simulink model "XMC_FFT2D_HLS_AIE"  (R2024a)
settings: Solver=VariableStepAuto  StartTime=0.0  StopTime=256*256*2  RelTol=1e-3
PreLoadFcn:
  | % display k space image & load arrays for
  | % simulation run
  | MRIDemo_PreloadFcn;
undefined symbols (not defined in the file): gray, None, S, vsva2197, xcvc1902
libraries: aieDSP x2, dspxfrm3 x2, dspsrcs4 x2, hlsBasic x1, simulink x1, vmcUtilities x1, aieUtilities x1
settings Model: Creator=mmi  LastModifiedBy=robg
settings SolverCC: AlgebraicLoopSolver=TrustRegion
settings DataIOCC: ReturnWorkspaceOutputs=off
settings DebuggingCC: UnconnectedInputMsg=warning  UnconnectedOutputMsg=warning  UnconnectedLineMsg=warning  ArithmeticOperatorsInVariantConditions=warning
settings ModelReferenceCC: EnableRefExpFcnMdlSchedulingChecks=on
settings SFSimCC: SimUseLocalCustomCode=off  CustomCodeUndefinedFunction=UseInterfaceOnly
settings RTWCC: RTWUseLocalCustomCode=off  GPUComputeCapability=3.5  DLArmComputeVersion=19.05
settings ConfigComp: CovBoundaryAbsTol=1.0e-5

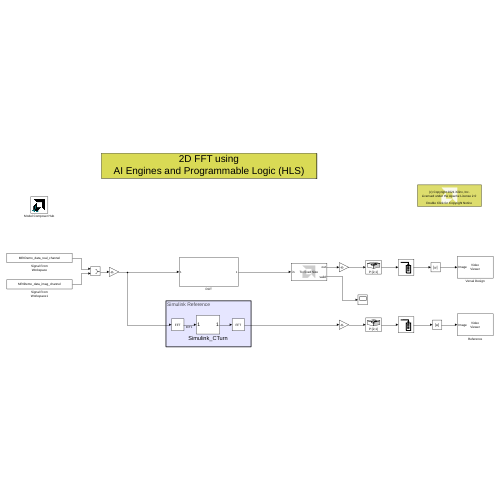
[thumbnail: Simulink's stored preview of the top-level diagram]
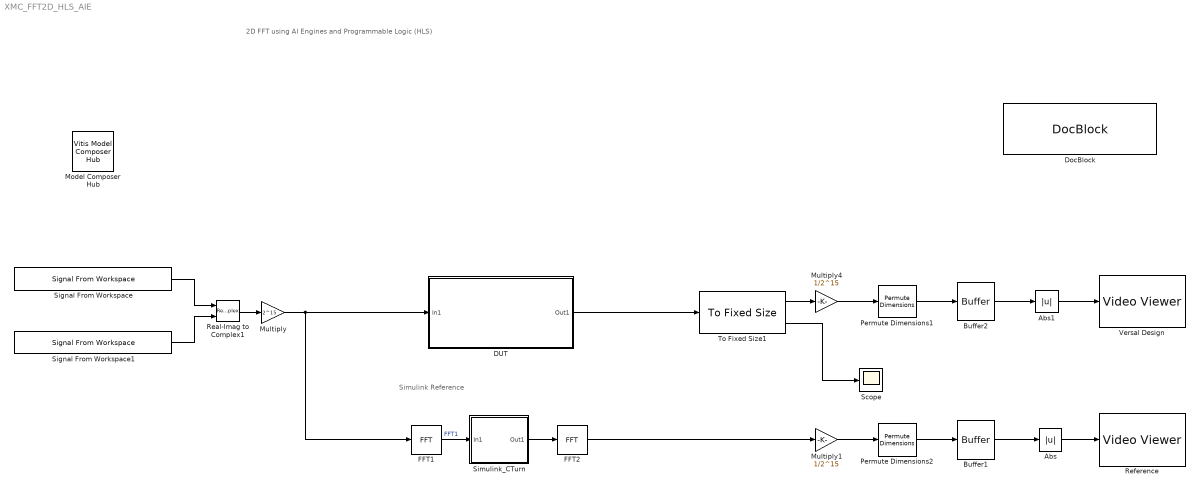
== system XMC_FFT2D_HLS_AIE ==
  note: Simulink Reference
  note: 2D FFT using
      | AI Engines and Programmable Logic (HLS)
  Abs : Abs  SaturateOnIntegerOverflow=off
  Abs1 : Abs  SaturateOnIntegerOverflow=off
  Buffer1 : Buffer  N=256  OutputFrames=off
  Buffer2 : Buffer  N=256  OutputFrames=off
  DUT : Subsystem
  DocBlock : simulink/Model-Wide Utilities/DocBlock  DocumentType=Text  mask(DocBlock){}
      content=|
      | ///////////////////////////////////////////////////////////////////////////
      | // Copyright 2021 Xilinx
      | //
      | // Licensed under the Apache License, Version 2.0 (the "License");
      | // you may not use this file except in compliance with the License.
      | // You may obtain a copy of the License at
      | //
      | // http://www.apache.org/licenses/LICENSE-2.0
      | //
      | // Unless required by applicable law or agreed to in writing, software
      | // distributed under the License is distributed on an "AS IS" BASIS,
      | // WITHOUT WARRANTIES OR CONDITIONS OF ANY KIND, either express or implied.
      | // See the License for the specific language governing permissions and
      | // limitations under the License.
      | ///////////////////////////////////////////////////////////////////////////
      mask Display:
      | xmcDrawBlockIcon();
      | disp(['{\fontsize{10pt}(c) Copyright 2021' ' Xilinx, Inc.}\newline \newline '],'texmode','on');
      | disp('{\fontsize{10pt}Licensed under the Apache License 2.0}','texmode','on');
      | disp('\newline \newline \newline{\fontsize{10pt}Double Click for Copyright Notice}','texmode','on');
  FFT1 : dspxfrm3/FFT  FFTImplementation=Auto  CompMethod=Table lookup  TableOpt=NEW  TableOptActive=Speed  BitRevOrder=off  Normalize=off  InheritFFTLength=on  FFTLength=64  WrapInput=on  roundingMode=Floor  overflowMode=off  firstCoeffDataTypeStr=Inherit: Same word length as input  firstCoeffLastDataTypeStr=Inherit: Same word length as input  prodOutputMode=Binary point scaling  prodOutputWordLength=32  prodOutputFracLength=0  prodOutputDataTypeStr=fixdt(1,32,0)  prodOutputLastDataTypeStr=fixdt(1,32,0)  accumMode=Binary point scaling  accumWordLength=48  accumFracLength=0  accumDataTypeStr=fixdt(1,48,0)  accumLastDataTypeStr=fixdt(1,48,0)  outputMode=Binary point scaling  outputWordLength=16  outputFracLength=0  outputDataTypeStr=fixdt(1,16,0)  outputMin=[]  outputMax=[]  outputLastDataTypeStr=fixdt(1,16,0)
  FFT2 : dspxfrm3/FFT  FFTImplementation=Auto  CompMethod=Table lookup  TableOpt=NEW  TableOptActive=Speed  BitRevOrder=off  Normalize=off  InheritFFTLength=on  FFTLength=64  WrapInput=on  roundingMode=Floor  overflowMode=off  firstCoeffDataTypeStr=Inherit: Same word length as input  firstCoeffLastDataTypeStr=Inherit: Same word length as input  prodOutputMode=Binary point scaling  prodOutputWordLength=32  prodOutputFracLength=0  prodOutputDataTypeStr=fixdt(1,32,0)  prodOutputLastDataTypeStr=fixdt(1,32,0)  accumMode=Binary point scaling  accumWordLength=48  accumFracLength=0  accumDataTypeStr=fixdt(1,48,0)  accumLastDataTypeStr=fixdt(1,48,0)  outputMode=Binary point scaling  outputWordLength=16  outputFracLength=0  outputDataTypeStr=fixdt(1,16,0)  outputMin=[]  outputMax=[]  outputLastDataTypeStr=fixdt(1,16,0)
  Model Composer Hub : vmcUtilities/Vitis Model Composer Hub  Tag=genX  CodeGeneration=off  SubsystemName=DUT  BlockHierPath=XMC_FFT2D_HLS_AIE/DUT  CompilationType=VitisCompilation  SubsystemType=DUTNode  AIEArrayConfig=Use entire AIE array  StartColumn=1  NumberOfColumns=1  TargetDirectory=./code  exportDesign=on  analyzeDesign=off  validateDesignOnHw=off  ExportType=Vitis Subsystem  IpVendor=xilinx.com  IpLibrary=hls  IpVersion=1.0  IpHWLanguage=Verilog  AieCompilerOptions={}  AieSimulatorOptions={}  CreateTestbench=off  TestbenchStackSize=10  RunRtlSim=off  RunCSim=off  RunAieSim=on  AieSimTimeout=50000  RunAieSimProfiling=off  LaunchVitisAnalyzer=off  PlotOutput=off  RunX86Sim=off  X86SimTimeout=10  GenHwImage=off  GenLibadfXo=on  GenHwValidationCode=on  PlatformType=Specify Platform  Platform=/proj/xbuilds/SWIP/9999.0_0818_1732/installs/lin64/2025.2/Vitis/base_platforms/xilinx_vck190_base_202520_1/xilinx_vck190_base_202520_1.xpfm  HwSystemType=Baremetal  HwValidationTarget=hw  ProjDevice=Versal VCK190 Evaluation Platform (xcvc1902-vsva2197-2MP-e-S)  ProjDevicePart=xcvc1902-vsva2197-2MP-e-S  AIEType=AIE  SamplePeriod=-1  ClockFrequency=200  DataPathParallelism=1  xilinxfamily=versalaicore  part=xcvc1902  speed=-2MP-e-S  package=vsva2197  directory=./netlist  testbench=off  incr_netlist=off  synthesis_tool=Vivado  clock_wrapper=Clock Enables  dbl_ovrd=According to Block Masks  dcm_input_clock_period=10  sysclk_period=10  simulink_period=1  eval_field=0  IPInfoJsonString="{\"DUTSubsystemName\":\"DUT\",\"HLSKernel\":{\"SubsystemName\":\"cturn2\",\"FpgaClockFreq\":\"200\",\"IPName\":\"cturn2\",\"IPLibrary\":\"hls\",\"TargetDirectory\":\"./code\",\"FreqHz\":\"200000000\",\"KernelFunction\":\"cturn2\"},\"SubsystemTag\":\"DUTNode\",\"AIESubsystem\":{\"SubsystemName\":\"aie_2dfft\",\"TargetDirectory\":\"./code\",\"AIEArrayConfig\":\"Use entire AIE array\",\"StartColumn\":\"1\",\"NumberOfColumns\":\"1\"}}"  LogFileName=/proj/xhdhdstaff5/sdegala/Head1/HEAD/VMC_2025_2_July/Examples/AIENGINE_plus_PL/AIE_HLS/FFT2D_HLS/code/model_composer.log  NThreads=4  IPConfigFile=/tmp/vmctmp-6835010160091439353/XMC_FFT2D_HLS_AIE_ipconfig.json
  Multiply : Gain  Gain=2^15  OutDataTypeStr=int16
  Multiply1 : Gain  Gain=1/2^15  OutDataTypeStr=single
  Multiply4 : Gain  Gain=1/2^15  OutDataTypeStr=single
  Permute Dimensions1 : PermuteDimensions
  Permute Dimensions2 : PermuteDimensions
  Real-Imag to Complex1 : RealImagToComplex
  Reference : VideoViewer  Description=Simulink MRI Display  colormapValue=gray(256)  FigPos=[147 767 631 287]
  Scope : Scope
  Signal From Workspace : dspsrcs4/Signal From Workspace  X=MRIDemo_data_real_channel  Ts=1  nsamps=256  OutputAfterFinalValue=Setting to zero  ignoreOrWarnInputAndFrameLengths=off  OutputFrames=off
  Signal From Workspace1 : dspsrcs4/Signal From Workspace  X=MRIDemo_data_imag_channel  Ts=1  nsamps=256  OutputAfterFinalValue=Setting to zero  ignoreOrWarnInputAndFrameLengths=off  OutputFrames=off
  Simulink_CTurn : Subsystem
  To Fixed Size1 : aieUtilities/To Fixed Size  Mode=Produce a valid output signal  OutputSize=256  CopyMethod=Buffer samples to form output  HasStatusOutput=off
  Versal Design : VideoViewer  Description=Simulink MRI Display  colormapValue=gray(256)  FigPos=[1055 882 683 266]
  wires:
  Signal From Workspace/1 -> Real-Imag to Complex1/1
  Signal From Workspace1/1 -> Real-Imag to Complex1/2
  FFT2/1 -> Multiply1/1
  Buffer1/1 -> Abs/1
  Permute Dimensions2/1 -> Buffer1/1
  Abs/1 -> Reference/1
  FFT1/1 -> Simulink_CTurn/1(In1)  "FFT1"
  Simulink_CTurn/1(Out1) -> FFT2/1
  Multiply/1 -> DUT/1(In1), FFT1/1
  Multiply1/1 -> Permute Dimensions2/1
  Real-Imag to Complex1/1 -> Multiply/1
  Buffer2/1 -> Abs1/1
  Abs1/1 -> Versal Design/1
  To Fixed Size1/1 -> Multiply4/1
  Permute Dimensions1/1 -> Buffer2/1
  Multiply4/1 -> Permute Dimensions1/1
  To Fixed Size1/2 -> Scope/1
  DUT/1(Out1) -> To Fixed Size1/1

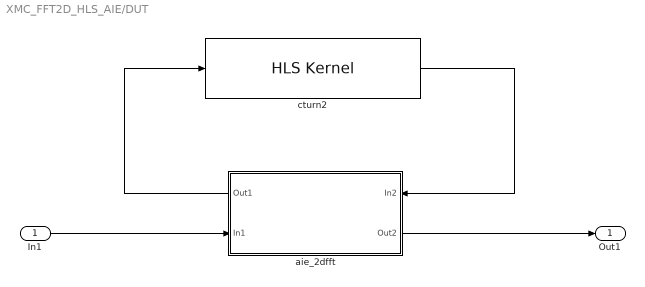
== system XMC_FFT2D_HLS_AIE/DUT ==
  In1 : Inport
  aie_2dfft : Subsystem
      settings: PortSchema="{\"entries\":[{\"content\":{\"sides\":[{\"content\":{\"connectorIds\":[\"Out2\",\"In1\"]},\"type\":\"ConnectorPlacement.EquallySpacedRectSide\",\"uuid\":\"79f05cc3-f11a-4cde-8fa1-dcc9430b22c8\"},{\"content\":{\"connectorIds\":[\"In2\",\"Out1\"],\"side\":\"RIGHT\"},\"type\":\"ConnectorPlacement.EquallySpacedRectSide\",\"uuid\":\"dca5e86a-9095-4cba-ba8f-7e749e0dbd7e\"},{\"content\":{\"connectorIds\":[],\"side\":\"TOP\"},\"type\":\"ConnectorPlacement.EquallySpacedRectSide\",\"uuid\":\"3830c194-8485-43cd-afe1-c92005d5a3f9\"}]},\"type\":\"ConnectorPlacement.EquallySpacedConnector\",\"uuid\":\"40ec3e32-3e8f-4730-8170-0d4e5db1f984\"}],\"packageUris\":[\"http://schema.mathworks.com/mf0/Connector/19700101\"],\"version\":\"1.0\"}"
  cturn2 : hlsBasic/HLS Kernel  PortNames={}  PortSerializedTypes={}  FunctionTemplateParamNames={}  FunctionTemplateParamKinds={}  FunctionTemplateParamTypes={}  FunctionTemplateParamValues={}  PortSynchronicities={'auto'; 'auto'}  PortSignalSizes={0.000000000000000000e+00; 2.560000000000000000e+02}  PortParameterValues={}  PortAttributesTable={ 'Input', 'vin', 'hls::stream< std::complex< int16 >, 0 > &', '', ''; 'Output', 'vout', 'hls::stream< std::complex< int16 >, 0 > &', '', '256' }  PortAttributesEnablement={'off', 'off', 'off', 'off', 'off';'off', 'off', 'off', 'off', 'on'}  PortParametersTable={}  SampleTime=-1  PortDirectionTable={'vin', 'hls::stream< std::complex< int16 >, 0 > &', 'Input', 'Port';'vout', 'hls::stream< std::complex< int16 >, 0 > &', 'Output', 'Port'}  FunctionTemplateParams={}  FunctionTemplateParamsEnables={}  FunctionTemplateParamsVisible=off  FunctionDeclTypeOptions=C[1 1]@t7@<empty>  PortDirectionTabVisible=on  ArgDirections={1.000000000000000000e+00; 2.000000000000000000e+00}  ArgInterfaceTypes={}  FunctionIndex=1  FormalArgDecls={'hls::stream< std::complex< int16 >, 0 > & vin', 'hls::stream< std::complex< int16 >, 0 > & vout'}  SimLibPath=''  FunctionTabVisible=on  FunctionDescription=void cturn2(hls::stream< std::complex< int16 >, 0 > & vin, hls::stream< std::complex< int16 >, 0 > & vout)  blockJsonConstraints=[]  deprecateConstraints=0  KernelHeaderFile=./src/cturn2.h  KernelFunction=cturn2  KernelFunctionSelect=<empty>  KernelSourceFile=./src/cturn2.cpp  KernelSearchPaths={}  PreProcOptions={}
  Out1 : Outport
  wires:
  cturn2/1 -> aie_2dfft/2(In2)
  aie_2dfft/2(Out1) -> cturn2/1
  In1/1 -> aie_2dfft/1(In1)
  aie_2dfft/1(Out2) -> Out1/1

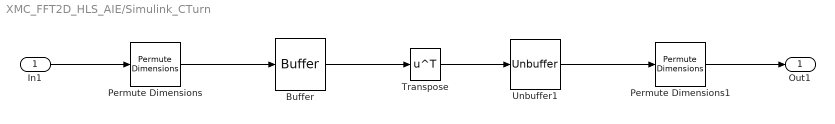
== system XMC_FFT2D_HLS_AIE/Simulink_CTurn ==
  In1 : Inport
  Buffer : Buffer  N=256  OutputFrames=off
  Permute Dimensions : PermuteDimensions
  Permute Dimensions1 : PermuteDimensions
  Transpose : Math  Operator=transpose  SignedPower=on
  Unbuffer1 : Unbuffer
  Out1 : Outport  VectorParamsAs1DForOutWhenUnconnected=off
  wires:
  Permute Dimensions/1 -> Buffer/1
  Transpose/1 -> Unbuffer1/1
  Buffer/1 -> Transpose/1
  In1/1 -> Permute Dimensions/1
  Unbuffer1/1 -> Permute Dimensions1/1
  Permute Dimensions1/1 -> Out1/1

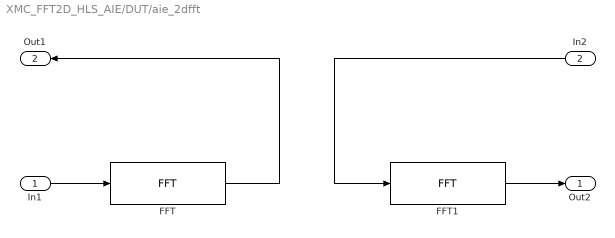
== system XMC_FFT2D_HLS_AIE/DUT/aie_2dfft ==
  In1 : Inport
  In2 : Inport  Port=2
  FFT : aieDSP/FFT  AIE_VARIANT=1  data_type=cint16  data_out_type=cint16  twiddle_type=cint16  point_size=256  input_window_size=256  shift_val=0  rnd_mode=Round to positive infinity  sat_mode=0-None  ssr=1  twiddle_mode=0  use_ssr_widget_kernels=off  casc_length=1  transform_fft_nifft=1  TP_API=0  TP_DYN_PT_SIZE=0  blockJsonConstraints=[]  blockJsonConstraintsInternal=[]  spec=vmc_fft.json  SerializedMaskParamNames=[]  SerializedMaskParamValues=[]  SerializedMaskParamVisibilities=[]  block_type=FFT  SerializedMaskParamDataypes=uint|typename|typename|typename|uint|uint|uint|uint|uint|uint|uint|uint|uint|uint|uint|uint  SerializedMaskParamEnumStrArr=0|0|0|0|0|0|0|Round to positive infinity,Round to negative infinity,Round symmetrical to infinity,Round symmetrical to zero,Round convergent to even,Round convergent to odd|0-None,1-Asymmetric,3-Symmetric|0|0|0|0|0|0|0  SerializedMaskParamEnumValArr=0|0|0|0|0|0|0|2,3,4,5,6,7|0,1,3|0|0|0|0|0|0|0  SerializedMaskParamVectorArr=0|0|0|0|0|0|0|0|0|0|0|0|0|0|0|0  SerializedMaskParamKeys=AIE_VARIANT|TT_DATA|TT_OUT_DATA|TT_TWIDDLE|TP_POINT_SIZE|TP_WINDOW_VSIZE|TP_SHIFT|TP_RND|TP_SAT|TP_PARALLEL_POWER|TP_TWIDDLE_MODE|TP_USE_WIDGETS|TP_CASC_LEN|TP_FFT_NIFFT|TP_API|TP_DYN_PT_SIZE
  FFT1 : aieDSP/FFT  AIE_VARIANT=1  data_type=cint16  data_out_type=cint16  twiddle_type=cint16  point_size=256  input_window_size=256  shift_val=0  rnd_mode=Round to positive infinity  sat_mode=0-None  ssr=1  twiddle_mode=0  use_ssr_widget_kernels=off  casc_length=1  transform_fft_nifft=1  TP_API=0  TP_DYN_PT_SIZE=0  blockJsonConstraints=[]  blockJsonConstraintsInternal=[]  spec=vmc_fft.json  SerializedMaskParamNames=[]  SerializedMaskParamValues=[]  SerializedMaskParamVisibilities=[]  block_type=FFT  SerializedMaskParamDataypes=uint|typename|typename|typename|uint|uint|uint|uint|uint|uint|uint|uint|uint|uint|uint|uint  SerializedMaskParamEnumStrArr=0|0|0|0|0|0|0|Round to positive infinity,Round to negative infinity,Round symmetrical to infinity,Round symmetrical to zero,Round convergent to even,Round convergent to odd|0-None,1-Asymmetric,3-Symmetric|0|0|0|0|0|0|0  SerializedMaskParamEnumValArr=0|0|0|0|0|0|0|2,3,4,5,6,7|0,1,3|0|0|0|0|0|0|0  SerializedMaskParamVectorArr=0|0|0|0|0|0|0|0|0|0|0|0|0|0|0|0  SerializedMaskParamKeys=AIE_VARIANT|TT_DATA|TT_OUT_DATA|TT_TWIDDLE|TP_POINT_SIZE|TP_WINDOW_VSIZE|TP_SHIFT|TP_RND|TP_SAT|TP_PARALLEL_POWER|TP_TWIDDLE_MODE|TP_USE_WIDGETS|TP_CASC_LEN|TP_FFT_NIFFT|TP_API|TP_DYN_PT_SIZE
  Out2 : Outport
  Out1 : Outport  Port=2
  wires:
  FFT/1 -> Out1/1
  FFT1/1 -> Out2/1
  In1/1 -> FFT/1
  In2/1 -> FFT1/1
